simulink model "simulink_tcp_try_1"  (R2019a)
settings: Solver=ode4  StartTime=0.0  StopTime=15  RelTol=1e-3  EnableMultiTasking=on
undefined symbols (not defined in the file): f
libraries: instrumentlib x2, mpclib x1, simulink x1
settings Model: Creator=alexh  LastModifiedBy=alexh
settings SolverCC: PositivePriorityOrder=on
settings OptimizationCC: EnhancedBackFolding=on  PassReuseOutputArgsAs=Individual arguments  MaxStackSize=64  OptimizeBlockOrder=speed  DifferentSizesBufferReuse=on  OptimizationCustomize=off
settings DebuggingCC: ParameterTunabilityLossMsg=error
settings HardwareCC: ProdBitPerPointer=32  ProdBitPerSizeT=32  ProdBitPerPtrDiffT=32  ProdLargestAtomicInteger=Long  ProdLargestAtomicFloat=Double  ProdWordSize=32  ProdLongLongMode=on  ProdHWDeviceType=ARM Compatible->ARM Cortex  UseEmbeddedCoderFeatures=off
settings SFSimCC: MATLABDynamicMemAlloc=off
settings RTWCC: SystemTargetFile=ert.tlc  HardwareBoard=Raspberry Pi  TLCOptions="-aInlineSetEventsForThisBaseRateFcn=TLC_FALSE -aSuppressMultiTaskScheduler=TLC_FALSE  -aRateBasedStepFcn=0"  TemplateMakefile=ert_default_tmf  GenerateReport=on  Toolchain=GNU GCC Raspberry Pi  BuildConfiguration=Faster Runs  IncludeHyperlinkInReport=on  LaunchReport=on  GenerateTraceInfo=on  GenerateTraceReport=on  GenerateTraceReportSl=on  GenerateTraceReportSf=on  GenerateTraceReportEml=on
settings CodeAppCC: ForceParamTrailComments=on  IgnoreCustomStorageClasses=off  OperatorAnnotations=on  SimulinkDataObjDesc=on  SFDataObjDesc=on  InsertBlockDesc=on
settings ERTTargetCC: SupportNonInlinedSFcns=on  SupportVariableSizeSignals=on

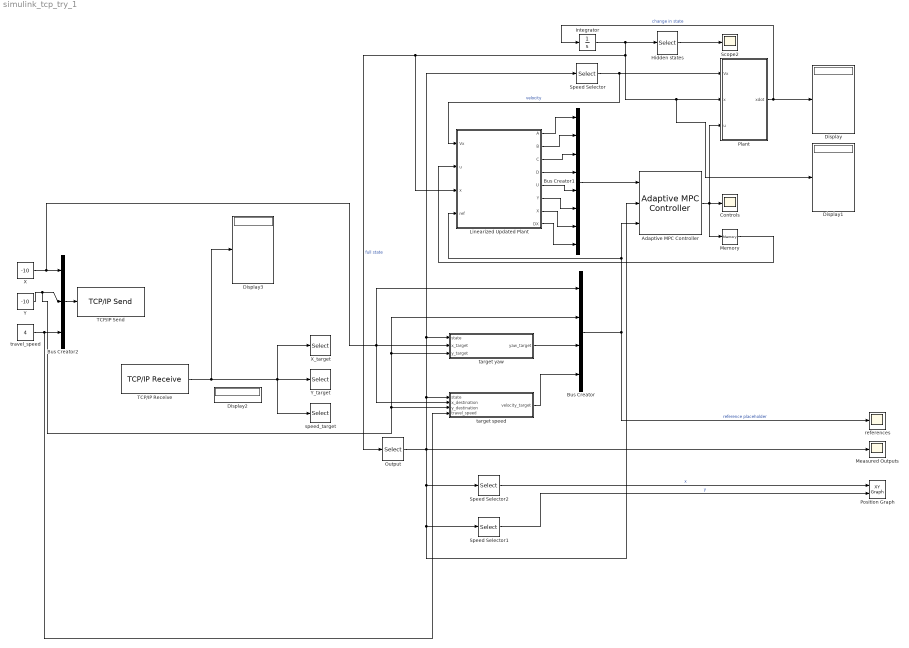
== system simulink_tcp_try_1 ==
  Adaptive MPC Controller : mpclib/Adaptive MPC Controller  SCDEnableBlockLinearizationSpecification=on  mpcobj=bycicle_mpc  enable_value=0  updateMPCinCallerWorkspace=on  md_inport=off  mv_inport=off  uref_inport=off  return_cost=off  return_mvseq=off  return_qpstatus=off  return_xseq=off  return_state=off  return_ovseq=off  state_inport=off  isltv_plant=off  umin_inport=off  umax_inport=off  ymin_inport=off  ymax_inport=off  cc_inport=off  ywt_inport=off  uwt_inport=off  duwt_inport=off  rhoeps_inport=off  pm_inport=off  MaximumP=10  HorizonChoice=FixedHorizon  BlockDataType=double  SampleTimeInherited=off  switch_inport=off
      settings: SourceProductName=MATLAB Runtime - Model Predictive Control Toolbox Addin  SourceProductBaseCode=Missing
  Bus Creator : BusCreator  Inputs=4
  Bus Creator1 : BusCreator  Inputs=8
  Bus Creator2 : BusCreator  Inputs=3
  Controls : Scope
  Display{,1..3} (4 alike) : Display
  Hidden states : Selector  InputPortWidth=6  IndexOptions=Index vector (dialog)  Indices=[4, 5]  OutputSizes=1
  Integrator : Integrator  InitialCondition=[0 0 0 0 0 0.01]
  Linearized Updated Plant : MATLAB Function  TreatAsAtomicUnit=on
  Measured Outputs : Scope
  Memory : Memory
  Output : Selector  InputPortWidth=6  IndexOptions=Index vector (dialog)  Indices=[1, 2, 3, 6]  OutputSizes=1
  "Plant " : MATLAB Function  TreatAsAtomicUnit=on
  Position Graph : simulink/Sinks/XY Graph  xmin=-15  xmax=15  ymin=-15  ymax=15  st=-1
  Scope2 : Scope
  Speed Selector : Selector  InputPortWidth=4  IndexOptions=Index vector (dialog)  Indices=[4]  OutputSizes=1
  Speed Selector1 : Selector  InputPortWidth=4  IndexOptions=Index vector (dialog)  Indices=[2]  OutputSizes=1
  Speed Selector2 : Selector  InputPortWidth=4  IndexOptions=Index vector (dialog)  Indices=[1]  OutputSizes=1
  TCP/IP Receive : instrumentlib/TCP//IP Receive  Host=localhost  Port=60389  DataSize="[1  3]"  EnableBlockingMode=on  Timeout=10  SampleTime=0.1  DataType=double  ByteOrder=BigEndian  ASCIIFormatting=%f,  Terminator=LF
      settings: SourceProductName=Instrument Control Toolbox
  TCP/IP Send : instrumentlib/TCP//IP Send  Host=localhost  Port=60389  EnableBlockingMode=on  Timeout=10  ByteOrder=BigEndian  TransferDelay=on
      settings: SourceProductName=Instrument Control Toolbox
  X : Constant  Value=-10
  X_target : Selector  InputPortWidth=3  IndexOptions=Index vector (dialog)  Indices=[1]  OutputSizes=1
  Y : Constant  Value=-10
  Y_target : Selector  InputPortWidth=3  IndexOptions=Index vector (dialog)  Indices=[2]  OutputSizes=1
  references : Scope
  speed_target : Selector  InputPortWidth=3  IndexOptions=Index vector (dialog)  Indices=[3]  OutputSizes=1
  target speed : MATLAB Function  TreatAsAtomicUnit=on
  target yaw : MATLAB Function  TreatAsAtomicUnit=on
  travel_speed : Constant  Value=4
  wires:
  "Plant "/1(xdot) -> Integrator/1, Display/1  "change in state"
  target speed/1(velocity_target) -> Bus Creator/4
  target yaw/1(yaw_target) -> Bus Creator/3
  Linearized Updated Plant/5(U) -> Bus Creator1/5
  Linearized Updated Plant/4(D) -> Bus Creator1/4
  Output/1 -> Speed Selector1/1, Adaptive MPC Controller/2, Speed Selector2/1, Speed Selector/1, target yaw/1(state), target speed/1(state), Measured Outputs/1
  Linearized Updated Plant/3(C) -> Bus Creator1/3
  Linearized Updated Plant/1(A) -> Bus Creator1/1
  Bus Creator1/1 -> Adaptive MPC Controller/1
  Linearized Updated Plant/2(B) -> Bus Creator1/2
  Linearized Updated Plant/8(DX) -> Bus Creator1/8
  Linearized Updated Plant/7(X) -> Bus Creator1/7
  Adaptive MPC Controller/1 -> "Plant "/3(u), Controls/1, Memory/1
  Memory/1 -> Linearized Updated Plant/2(u)
  Speed Selector2/1 -> Position Graph/1  "x"
  Bus Creator/1 -> Adaptive MPC Controller/3, Linearized Updated Plant/4(ref), references/1  "reference placeholder"
  Speed Selector1/1 -> Position Graph/2  "y"
  Hidden states/1 -> Scope2/1
  travel_speed/1 -> target speed/4(travel_speed), Bus Creator2/3
  Linearized Updated Plant/6(Y) -> Bus Creator1/6
  Integrator/1 -> Linearized Updated Plant/3(x), Output/1, Display1/1, "Plant "/2(x), Hidden states/1  "full state"
  Y/1 -> target yaw/3(y_target), Bus Creator/2, target speed/3(y_destination), Bus Creator2/2
  Speed Selector/1 -> "Plant "/1(Vx), Linearized Updated Plant/1(Vx)  "velocity"
  X/1 -> target speed/2(x_destination), Bus Creator/1, target yaw/2(x_target), Bus Creator2/1
  TCP/IP Receive/1 -> Display3/1, speed_target/1, X_target/1, Y_target/1
  ? -> Display2/1
  Bus Creator2/1 -> TCP/IP Send/1

== matlab function simulink_tcp_try_1/Linearized Updated Plant ==
  data: Vx input; u input; A output; x input; B output; C output; D output; U output; Y output; X output; DX output; ref input
function [A,B,C,D,U,Y,X,DX] = fcn(Vx,u,x, ref)
% Sample time
Ts = 0.1;

% Model parameters
%m = 1575;
%iz = 2875;
%lf = 1.2;
%lr = 1.6;
%cf = 19000;
%cr = 33000;
m = 125;
iz = 287;
lf = 0.6;
lr = 0.6;
cf = 190;
cr = 330;

if (Vx<0.1)
       Vx = 0.1;
end

% we have to tweak the system a bit to make it realize altering the 
% speed can do something for reaching the destination
if (x(2)<ref(2))
    speed_influence = 0.1;
else
    speed_influence = -0.1;
end

% Continuous-time model
Ac = [0, 0, -Vx, 0, -1, Vx;
       0, 0, Vx, 0, 1, speed_influence;
       0, 0, 0, 1, 0, 0;
       0, 0, 0, -(2*cf*lf^2+2*cr*lr^2)/iz/Vx, -(2*cf*lf-2*cr*lr)/iz/Vx, 0;
       0, 0, 0,  -Vx-(2*cf*lf-2*cr*lr)/m/Vx, -(2*cf+2*cr)/m/Vx, 0;
       0, 0, 0, 0, 0, -.1];
   
 Bc = [0, 0, 0, 2*cf*lf/iz, 2*cf/m, 0;
        0, 0, 0, 0, 0, 1]';
 
 % Position, Yaw, Speed
 Cc = [1, 0, 0, 0, 0, 0;
        0, 1, 0, 0, 0, 0;
        0, 0, 1, 0, 0, 0;
        0, 0, 0, 0, 0, 1];
    
 Dc = zeros(4, 2);

% Generate discrete-time model
nx = size(Ac,1);
nu = size(Bc,2);
M = expm([[Ac Bc]*Ts; zeros(nu,nx+nu)]);
A = M(1:nx,1:nx);
B = M(1:nx,nx+1:nx+nu);
C = Cc;
D = Dc;

% Nominal conditions for discrete-time plant
X = x';
U = u';
Y = (C*x + D*u)';
DX = (A*x+B*u-x)';      % did this fix, might be wrong

== matlab function simulink_tcp_try_1/Plant  ==
  data: Vx input; x input; u input; xdot output
function xdot = fcn(Vx,x,u)

if (Vx<0.1)
    Vx=0.1;
end

% Model parameters
m = 125;
iz = 287;
lf = 0.6;
lr = 0.6;
cf = 190;
cr = 330;

sin_yaw = sin(x(3));
cos_yaw = cos(x(3));


% Continuous-time model
% Continuous-time model
Ac = [0, 0, 0, 0, 0, cos_yaw;
       0, 0, 0, 0, 0, sin_yaw;
       0, 0, 0, 1, 0, 0;
       0, 0, 0, -(2*cf*lf^2+2*cr*lr^2)/iz/Vx, -(2*cf*lf-2*cr*lr)/iz/Vx, 0;
       0, 0, 0,  -Vx-(2*cf*lf-2*cr*lr)/m/Vx, -(2*cf+2*cr)/m/Vx, 0;
       0, 0, 0, 0, 0, -.1];
   
 Bc = [0, 0, 0, 2*cf*lf/iz, 2*cf/m, 0;
        0, 0, 0, 0, 0, 1]';

xdot = Ac*x + Bc*u;

== matlab function simulink_tcp_try_1/target yaw ==
  data: state input; yaw_target output; x_target input; y_target input
function yaw_target = fcn(state, x_target, y_target)

% Rearange data
position = [state(1) state(2)];
position_target = [x_target, y_target]';
x = state(1);
y = state(2);
yaw = state(3);

% Calculate target yaw
yaw_target = atan((abs(y) - abs(y_target)) / (abs(x) - abs(x_target)));
if x - x_target > 0 && y - y_target < 0         % 2nd q
    yaw_target = pi - yaw_target;
elseif x - x_target > 0 && y - y_target > 0     % 3rd q
    yaw_target = -pi + yaw_target;
elseif x - x_target < 0 && y - y_target > 0     % 4th q
    yaw_target = -yaw_target;
end

% Adjust so we actually take shortest doff
yaw_diff = acos((position * position_target) / (norm(position) * norm(position_target)));

%if ((yaw + yaw_diff) > pi) && (yaw > yaw_target)
%    yaw_target = yaw_target + 2*pi;
%elseif((yaw - yaw_diff) < -pi) && (yaw < yaw_target)
%    yaw_target = yaw_target - 2*pi;
%end

if yaw_diff < pi
    if yaw_target < 0 && yaw > 0
        %yaw_target = yaw_target + 2*pi;
    end
    if yaw_target > 0 && yaw < 0
        %yaw_target = yaw_target - 2*pi;
    end    
end

% Avoid strong steering impulses when close to destination 
if (x_target-x)^2 + (y_target-y)^2 < 1
    yaw_target = 0;
end

== matlab function simulink_tcp_try_1/target speed ==
  data: state input; velocity_target output; x_destination input; y_destination input; travel_speed input
function velocity_target = fcn(state, x_destination, y_destination, travel_speed)

% Rearange data
position = [state(1) state(2)];
position_target = [x_destination, y_destination];

% Calculate delta position
delta_position = position - position_target;

distance_to_travel = norm(delta_position);

velocity_target = min(travel_speed, distance_to_travel/2);
